simulink model "Privodslx"  (R2022a)
settings: Solver=VariableStepAuto  StartTime=0.0  StopTime=inf  FixedStep=0.01  RelTol=1e-3
undefined symbols (not defined in the file): diff, eul2tform, get, hot, Levenberg, Marquardt, maxWaypoints, q0, traectory, trvec2tform, ts, waypointTimes, X, Y, Z
libraries: sm_lib x250, nesl_utility x51, trajExampleUtils x23, robotcorelib x19, robotmaniplib x5, Contact_Forces_Lib x1, dspobslib x1
(part 1 of 6)
settings Model: Creator=tystr  LastModifiedBy=tystr
settings SolverCC: AlgebraicLoopSolver=TrustRegion
settings DebuggingCC: ReadBeforeWriteMsg=DisableAll  WriteAfterWriteMsg=DisableAll  WriteAfterReadMsg=DisableAll  MultiTaskDSMMsg=none  UnconnectedInputMsg=warning  UnconnectedOutputMsg=warning  UnconnectedLineMsg=warning  SFMachineParentedDataDiag=warning
settings SFSimCC: CustomCodeUndefinedFunction=UseInterfaceOnly
settings RTWCC: DLArmComputeVersion=19.05
settings ExplorerConfigSet: InternalSimMechanicsExplorerSettings="<ExplorerConfiguration><canonicalview>default</canonicalview><AnimationSetting><BasePlaybackSpeed>1.0</BasePlaybackSpeed><PlaybackSpeedFactor>1.0</PlaybackSpeedFactor></AnimationSetting><TilePanel><TileInfo><Tiles Columns=\"1\" Count=\"1\" Rows=\"1\"><Column Weight=\"1\"/><Row Weight=\"1\"/><Tile Height=\"1\" Width=\"1\" X=\"0\" Y=\"0\"/></Tiles></TileInfo><SceneInfo><SceneViewer><BGColor><R>0.800000011920928955</R><G>0.800000011920928955</G><B>0.800000011920928955</B></BGColor><Camera><DoPerspective>off</DoPerspective><Position><X>0.581172870773565831</X><Y>-0.777808712780073574</Y><Z>0.308286162888697479</Z></Position><Center><X>0.305915452038245772</X><Y>0.176306748607351294</Y><Z>0.190400456491913256</Z></Center><Up><X>-0.216141355262336798</X><Y>0.0580651955211244353</Y><Z>0.974633955705655919</Z></Up><ViewLimDist>1</ViewLimDist><YLim>0.905328153776305378</YLim><XLim>1.29865056944726809</XLim></Camera></SceneViewer></SceneInfo></TilePanel><MechEditorPanel><Cameras><Camera><Id>Camera1</Id><Value><Name>Camera1</Name><NativeCamera><PositionTrackingFeature>UR1.tool0.F.frame</PositionTrackingFeature><CenterTrackingFeature>UR1.tool0.F.frame</CenterTrackingFeature><UpVectorTrackingFeature>UR1.tool0.F.frame</UpVectorTrackingFeature><CenterTrackingOrigin>off</CenterTrackingOrigin><CenterTrackingDirection>+Z</CenterTrackingDirection><UpVectorTrackingDirection>-X</UpVectorTrackingDirection></NativeCamera></Value></Camera></Cameras><GfxPanelCameraMap/><VideoCreator><PlaybackSpeedRatio>1.0</PlaybackSpeedRatio><FrameRate>60</FrameRate><VideoFormat>MPEG-4</VideoFormat><FrameSize>[1920 1080]</FrameSize></VideoCreator></MechEditorPanel></ExplorerConfiguration>"

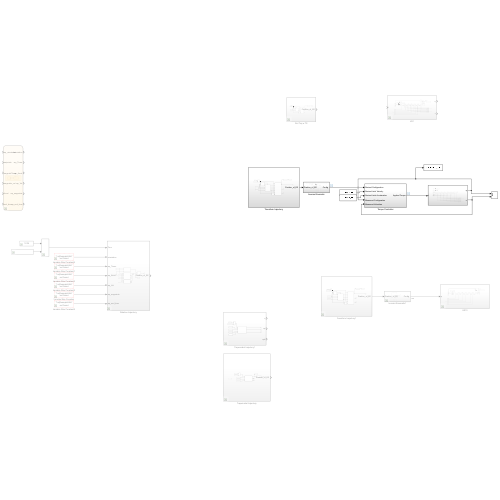
[thumbnail: Simulink's stored preview of the top-level diagram]
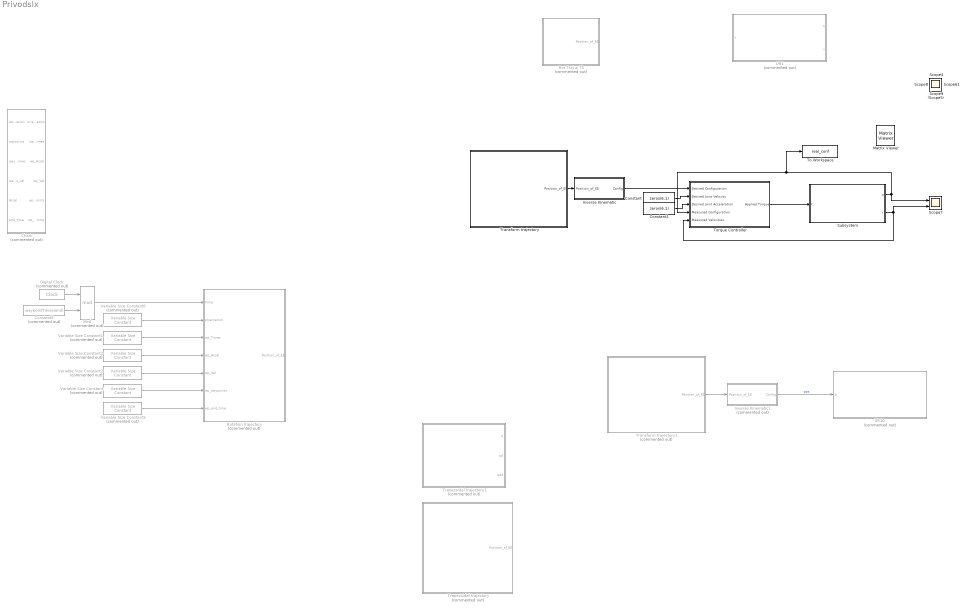
== system Privodslx ==
  Chart : Stateflow chart  Commented=on  TreatAsAtomicUnit=on
      settings: PortSchema="{\"entries\":[{\"content\":{\"sides\":[{\"content\":{\"connectorIds\":[\"In4\",\"In2\",\"In1\",\"In3\",\"In5\",\"In6\"]},\"type\":\"ConnectorPlacement.EquallySpacedRectSide\",\"uuid\":\"199a3ae9-d570-4542-b92b-f36511b0c15c\"},{\"content\":{\"connectorIds\":[\"Out1\",\"Out2\",\"Out3\",\"Out4\",\"Out5\",\"Out6\"],\"side\":\"RIGHT\"},\"type\":\"ConnectorPlacement.EquallySpacedRectSide\",\"uuid\":\"03e9b347-4596-49f5-8d91-254a4ca3c338\"},{\"content\":{\"connectorIds\":[],\"side\":\"TOP\"},\"type\":\"ConnectorPlacement.EquallySpacedRectSide\",\"uuid\":\"99359905-edef-4f33-b514-45af203258c0\"},{\"content\":{\"connectorIds\":[],\"side\":\"HIDDEN\"},\"type\":\"ConnectorPlacement.EquallySpacedRectSide\",\"uuid\":\"67583bbf-e95c-431d-a69b-7f52f21df5ab\"}]},\"type\":\"ConnectorPlacement.EquallySpacedConnector\",\"uuid\":\"4447fce3-df88-4ff0-a93e-6e37d8f328a3\"}],\"packageUris\":[\"http://schema.mathworks.com/mf0/Connector/R2020b\"],\"version\":\"1.0\"}"
  Constant : Constant  Value=zeros(6,1)  SampleTime=0.01
  Constant1 : Constant  Value=zeros(6,1)  SampleTime=0.01
  Constant5 : Constant  Commented=on  Value=waypointTimes(end)
  Digital Clock : DigitalClock  Commented=on  SampleTime=ts
  Inverse Kinematic : Subsystem
  Inverse Kinematic1 : Subsystem  Commented=on
  Mod : Math  Commented=on  Operator=mod  SignedPower=on
  Rot Traj w TS : Subsystem  Commented=on
  Rotation trajectory : Subsystem  Commented=on
  Scope7 : Scope  NumInputPorts=2
  Subsystem : Subsystem
  To Workspace : ToWorkspace  VariableName=real_conf  SaveFormat=Timeseries  SampleTime=-1
  Torque Controller : Subsystem
  Transform trajectory : Subsystem
  Transform trajectory1 : Subsystem  Commented=on
  Trapezoidal trajectory : Subsystem  Commented=on
  Trapezoidal trajectory1 : Subsystem  Commented=on
  UR1 : Subsystem  Commented=on
  UR10 : Subsystem  Commented=on
  Variable Size Constant : trajExampleUtils/Variable Size Constant  Commented=on  val=waypoints  maxSize=[3,maxWaypoints]  Ts=ts  SSRTWFcnClass=[]
  Variable Size Constant1 : trajExampleUtils/Variable Size Constant  Commented=on  val=waypointTimes  maxSize=[1,maxWaypoints]  Ts=ts  SSRTWFcnClass=[]
  Variable Size Constant2 : trajExampleUtils/Variable Size Constant  Commented=on  val=waypointVels  maxSize=[3,maxWaypoints]  Ts=ts  SSRTWFcnClass=[]
  Variable Size Constant3 : trajExampleUtils/Variable Size Constant  Commented=on  val=waypointAccels  maxSize=[3,maxWaypoints]  Ts=ts  SSRTWFcnClass=[]
  Variable Size Constant5 : trajExampleUtils/Variable Size Constant  Commented=on  val=repmat(diff(waypointTimes),[3 1])  maxSize=[3,maxWaypoints-1]  Ts=ts  SSRTWFcnClass=[]
  Variable Size Constant6 : trajExampleUtils/Variable Size Constant  Commented=on  val=orientations  maxSize=[3,maxWaypoints]  Ts=ts  SSRTWFcnClass=[]
  Matrix Viewer : dspobslib/Matrix Viewer  IOType=viewer  ImageParams=off  CMapStr=hot(256)  AxisColorbar=on  AxisParams=off  AxisOrigin=Upper left corner  AxisTickMode=Auto  XTickRange=[0 1]  YTickRange=[0 1]  XLabel=X-axis  YLabel=Y-axis  ZLabel=Z-axis  FigPos=get(0,'defaultfigureposition')  AxisZoom=off
      settings: SourceProductName=DSP System Toolbox  YMin=-1.0  YMax=1.0
  Scope{,1..6,8..11} (11 alike) : Scope
  wires:
  Transform trajectory1/1("Position_of_EE ") -> Inverse Kinematic1/1("Position_of_EE ")
  Inverse Kinematic1/1("Config ") -> UR10/1(q)  "pos"
  Constant1/1 -> Torque Controller/3(Desired Joint Acceleration)
  Digital Clock/1 -> Mod/1
  Constant5/1 -> Mod/2
  Mod/1 -> Rotation trajectory/1(Time)
  Variable Size Constant6/1 -> Rotation trajectory/2(orientation)
  Variable Size Constant/1 -> Rotation trajectory/6(wp_waypoints)
  Variable Size Constant1/1 -> Rotation trajectory/3(wp_Times)
  Variable Size Constant2/1 -> Rotation trajectory/5(wp_Vel)
  Variable Size Constant3/1 -> Rotation trajectory/4(wp_Accel)
  Variable Size Constant5/1 -> Rotation trajectory/7(wp_end_time)
  Constant/1 -> Torque Controller/2(Desired Joint Velocity)
  Transform trajectory/1("Position_of_EE ") -> Inverse Kinematic/1("Position_of_EE ")
  Subsystem/1(q) -> Scope7/1, To Workspace/1, Torque Controller/4(Measured Configuration)
  Subsystem/2(v) -> Torque Controller/5(Measured Velocities), Scope7/2
  Torque Controller/1(Applied Torque) -> Subsystem/1(t)
  Inverse Kinematic/1("Config ") -> Torque Controller/1(Desired Configuration)

== system Privodslx/Inverse Kinematic ==
  "Position_of_EE " : Inport  SampleTime=ts
  Bus Selector : BusSelector  Commented=on  OutputSignals=Iterations,PoseErrorNorm,ExitFlag,Status
  Constant : Constant  Value=[1,1,1,1,1,1]
  Delay : Delay  DelayLength=1  InitialCondition=q0  SampleTime=ts
  Display{3..6} (4 alike) : Display  Commented=on
  Inverse Kinematics : robotmaniplib/Inverse Kinematics  RigidBodyTree=robot  EndEffector=tool0  ShowInfo=on  SolverName=Levenberg-Marquardt  EnforceJointLimits=on  MaxIterations=1500  MaxTime=10  GradientTolerance=1e-7  SolutionTolerance=1e-6  StepTolerance=1e-14  ErrorChangeTolerance=1e-12  UseErrorDamping=on  DampingBias=0.0025  SimulateUsing=Interpreted execution
  To Workspace : ToWorkspace  VariableName=config  SaveFormat=Timeseries  SampleTime=-1
  To Workspace1 : ToWorkspace  VariableName=info  SaveFormat=Timeseries  SampleTime=-1
  "Config " : Outport  SampleTime=ts  VectorParamsAs1DForOutWhenUnconnected=off
  wires:
  Bus Selector/3 -> Display5/1  "<ExitFlag>"
  Inverse Kinematics/1 -> Delay/1, To Workspace/1, "Config "/1
  Bus Selector/4 -> Display6/1  "<Status>"
  Inverse Kinematics/2 -> To Workspace1/1
  Bus Selector/2 -> Display4/1  "<PoseErrorNorm>"
  "Position_of_EE "/1 -> Inverse Kinematics/1
  Constant/1 -> Inverse Kinematics/2
  Bus Selector/1 -> Display3/1  "<Iterations>"
  Delay/1 -> Inverse Kinematics/3

== system Privodslx/Inverse Kinematic1 ==
  "Position_of_EE " : Inport
  Bus Selector : BusSelector  Commented=on  OutputSignals=Iterations,PoseErrorNorm,ExitFlag,Status
  Constant : Constant  Value=[1,1,1,1,1,1]
  Delay : Delay  DelayLength=1  InitialCondition=zeros(6,1)
  Display : Display
  Display{3..6} (4 alike) : Display  Commented=on
  Inverse Kinematics1 : robotmaniplib/Inverse Kinematics  RigidBodyTree=robot  EndEffector=tool0  ShowInfo=on  SolverName=Levenberg-Marquardt  EnforceJointLimits=off  MaxIterations=1500  MaxTime=10  GradientTolerance=1e-7  SolutionTolerance=1e-6  StepTolerance=1e-14  ErrorChangeTolerance=1e-12  UseErrorDamping=on  DampingBias=0.0025  SimulateUsing=Interpreted execution
  Scope : Scope
  To Workspace : ToWorkspace  VariableName=config  SaveFormat=Timeseries  SampleTime=-1
  To Workspace1 : ToWorkspace  VariableName=info  SaveFormat=Timeseries  SampleTime=-1
  "Config " : Outport  VectorParamsAs1DForOutWhenUnconnected=off
  wires:
  Bus Selector/1 -> Display3/1  "<Iterations>"
  Constant/1 -> Inverse Kinematics1/2
  "Position_of_EE "/1 -> Inverse Kinematics1/1, Display/1
  Delay/1 -> Inverse Kinematics1/3
  Bus Selector/2 -> Display4/1  "<PoseErrorNorm>"
  Inverse Kinematics1/2 -> To Workspace1/1
  Bus Selector/4 -> Display6/1  "<Status>"
  Inverse Kinematics1/1 -> Delay/1, "Config "/1, Scope/1, To Workspace/1
  Bus Selector/3 -> Display5/1  "<ExitFlag>"

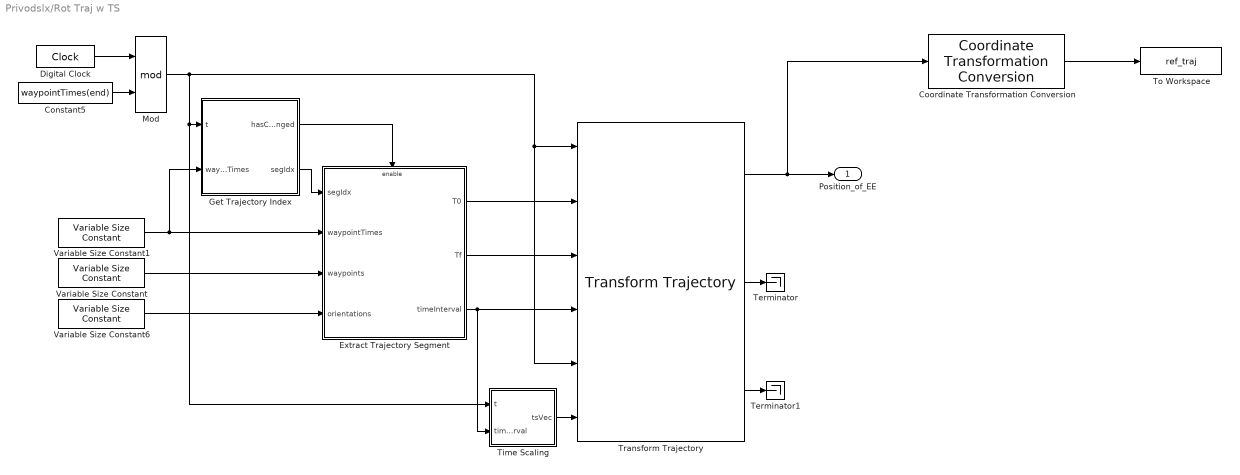
== system Privodslx/Rot Traj w TS ==
  Constant5 : Constant  Value=waypointTimes(end)
  Coordinate Transformation Conversion : robotcorelib/Coordinate Transformation Conversion  InputRepresentation=Homogeneous Transformation  InputEulerSequence=ZYX  ShowTrVecInputPort=on  OutputRepresentation=Translation Vector  OutputEulerSequence=ZYX  ShowTrVecOutputPort=on  SimulateUsing=Interpreted execution
      settings: SourceProductBaseCode=RO,NV,RR,UV
  Digital Clock : DigitalClock  SampleTime=ts
  Extract Trajectory Segment : Subsystem
  Get Trajectory Index : MATLAB Function  TreatAsAtomicUnit=on
  Mod : Math  Operator=mod  SignedPower=on
  Terminator : Terminator
  Terminator1 : Terminator
  Time Scaling : Subsystem
  To Workspace : ToWorkspace  VariableName=ref_traj  SaveFormat=Timeseries  SampleTime=-1
  Transform Trajectory : robotcorelib/Transform Trajectory  WaypointSource=External  T0=trvec2tform( [ 1, 10, -1 ] )  TF=eul2tform( [ 0, pi, pi / 2 ] )  TimeInterval=[ 2, 3 ]  CustomTimeScaling=on  ParameterSource=External  TSTime=2:0.1:3  TimeScaling=[ 0:0.1:1; ones( 1, 11 ); zeros( 1, 11 ) ]  SimulateUsing=Interpreted execution
      settings: SourceProductBaseCode=RO,NV,RR,UV
  Variable Size Constant : trajExampleUtils/Variable Size Constant  val=waypoints  maxSize=[3,maxWaypoints]  Ts=-1
  Variable Size Constant1 : trajExampleUtils/Variable Size Constant  val=waypointTimes  maxSize=[1,maxWaypoints]  Ts=-1
  Variable Size Constant6 : trajExampleUtils/Variable Size Constant  val=orientations  maxSize=[3,maxWaypoints]  Ts=-1
  "Position_of_EE " : Outport
  wires:
  Variable Size Constant1/1 -> Extract Trajectory Segment/2(waypointTimes), Get Trajectory Index/2(waypointTimes)
  Transform Trajectory/2 -> Terminator/1
  Variable Size Constant6/1 -> Extract Trajectory Segment/4(orientations)
  Time Scaling/1(tsVec) -> Transform Trajectory/6
  Mod/1 -> Transform Trajectory/1, Transform Trajectory/5, Time Scaling/1(t), Get Trajectory Index/1(t)
  Extract Trajectory Segment/3(timeInterval) -> Transform Trajectory/4, Time Scaling/2(timeInterval)
  Extract Trajectory Segment/2(Tf) -> Transform Trajectory/3
  Get Trajectory Index/2(segIdx) -> Extract Trajectory Segment/1(segIdx)
  Extract Trajectory Segment/1(T0) -> Transform Trajectory/2
  Get Trajectory Index/1(hasChanged) -> Extract Trajectory Segment/Enable
  Transform Trajectory/3 -> Terminator1/1
  Variable Size Constant/1 -> Extract Trajectory Segment/3(waypoints)
  Digital Clock/1 -> Mod/1
  Constant5/1 -> Mod/2
  Transform Trajectory/1 -> Coordinate Transformation Conversion/1, "Position_of_EE "/1
  Coordinate Transformation Conversion/1 -> To Workspace/1

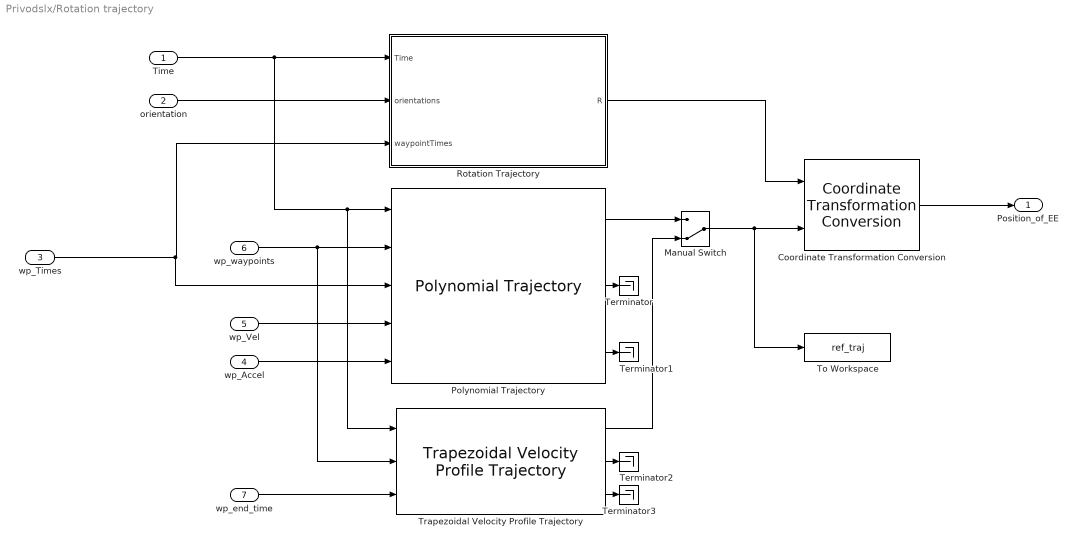
== system Privodslx/Rotation trajectory ==
  Time : Inport
  orientation : Inport  Port=2
  wp_Times : Inport  Port=3
  wp_Accel : Inport  Port=4
  wp_Vel : Inport  Port=5
  wp_waypoints : Inport  Port=6
  wp_end_time : Inport  Port=7
  Coordinate Transformation Conversion : robotcorelib/Coordinate Transformation Conversion  InputRepresentation=Quaternion  InputEulerSequence=ZYX  ShowTrVecInputPort=on  OutputRepresentation=Homogeneous Transformation  OutputEulerSequence=ZYX  ShowTrVecOutputPort=on  SimulateUsing=Interpreted execution
      settings: SourceProductBaseCode=RO,NV,RR,UV
  Manual Switch : ManualSwitch  CurrentSetting=0
  Polynomial Trajectory : robotcorelib/Polynomial Trajectory  WaypointSource=External  Waypoints=[ 0, 2, 1, 5, 0; -1, 3, 1, 4, 4 ]  TimePoints=[ 0, 1, 2, 3, 4 ]  TimeInterval=[ 1, 4 ]  Method=Quintic Polynomial  ParameterSource=External  VelocityBoundaryCondition=zeros( 2, 5 )  AccelerationBoundaryCondition=zeros( 2, 5 )  SimulateUsing=Interpreted execution
      settings: SourceProductBaseCode=RO,NV,RR,UV
  Rotation Trajectory : Subsystem
  Terminator{,1..3} (4 alike) : Terminator
  To Workspace : ToWorkspace  VariableName=ref_traj  SaveFormat=Timeseries  SampleTime=-1
  Trapezoidal Velocity Profile Trajectory : robotcorelib/Trapezoidal Velocity Profile Trajectory  WaypointSource=External  Waypoints=[ 0, -0.5, -1; 0, 0.5, 1 ]  NumParams=1  Parameter1=End Time  Parameter2=End Time  ParameterSource=External  PeakVelocity=[ 1; 1; 1 ]  Acceleration=[ 1; 2 ]  EndTime=[ 1; 1; 1 ]  AccelTime=[ 1; 2 ]  SimulateUsing=Interpreted execution
      settings: SourceProductBaseCode=RO,NV,RR,UV
  "Position_of_EE " : Outport  SampleTime=ts
  wires:
  Manual Switch/1 -> To Workspace/1, Coordinate Transformation Conversion/2
  Polynomial Trajectory/1 -> Manual Switch/1
  Trapezoidal Velocity Profile Trajectory/2 -> Terminator2/1
  Rotation Trajectory/1(R) -> Coordinate Transformation Conversion/1
  Trapezoidal Velocity Profile Trajectory/3 -> Terminator3/1
  Trapezoidal Velocity Profile Trajectory/1 -> Manual Switch/2
  Polynomial Trajectory/3 -> Terminator1/1
  Polynomial Trajectory/2 -> Terminator/1
  Coordinate Transformation Conversion/1 -> "Position_of_EE "/1
  Time/1 -> Trapezoidal Velocity Profile Trajectory/1, Polynomial Trajectory/1, Rotation Trajectory/1(Time)
  orientation/1 -> Rotation Trajectory/2(orientations)
  wp_Times/1 -> Polynomial Trajectory/3, Rotation Trajectory/3(waypointTimes)
  wp_Accel/1 -> Polynomial Trajectory/5
  wp_Vel/1 -> Polynomial Trajectory/4
  wp_waypoints/1 -> Trapezoidal Velocity Profile Trajectory/2, Polynomial Trajectory/2
  wp_end_time/1 -> Trapezoidal Velocity Profile Trajectory/3

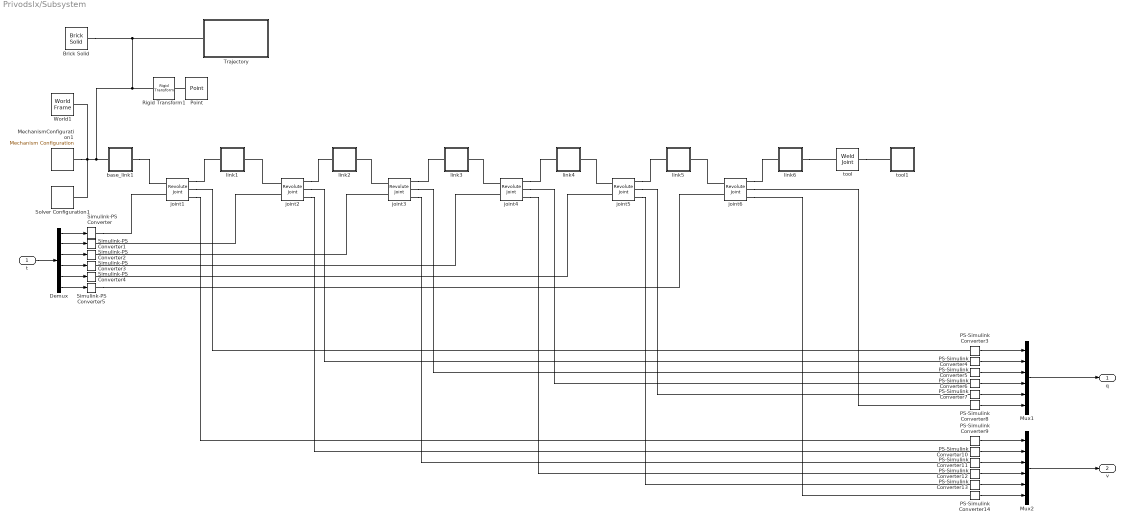
== system Privodslx/Subsystem ==
  t : Inport  SampleTime=ts
  Brick Solid : sm_lib/Body Elements/Brick Solid  GraphicAmbientColor=[0.15 0.15 0.15 1.0]  BasedOnType=Density  BrickDimensions=[1.5 1.5 0.01]  BrickDimensionUnits=m  CenterOfMass=[0 0 0]  CenterOfMassUnits=m  GraphicDiffuseColor=[0.5019608 0.72156864 0.3019608]  Density=1000  DensityUnits=kg/m^3  DoExposeReferenceFrame=on  GraphicEmissiveColor=[0.0 0.0 0.0 1.0]  ExportEntireGeometry=off  SerializedFrames=<Frames/>  MarkerShape=Sphere  MarkerSize=10  GraphicType=FromGeometry  InertiaType=CalculateFromGeometry  Mass=1  MassUnits=kg  MomentsOfInertia=[1 1 1]  MomentsOfInertiaUnits=kg*m^2  GraphicOpacity=1.0  ProductsOfInertia=[0 0 0]  ProductsOfInertiaUnits=kg*m^2  GraphicShininess=75  GraphicSpecularColor=[0.5 0.5 0.5 1.0]  GraphicVisPropType=SimpleVisualProperties
  Demux : Demux  Outputs=6
  MechanismConfiguration1 : sm_lib/Utilities/Mechanism Configuration  UniformGravity=Constant  GravityVector=[0 0 -9.80665]  GravityUnits=m/s^2  LinearizationDelta=0.001  JointModeTransitionNonlinearIterations=2
  Mux1 : Mux  Inputs=6
  Mux2 : Mux  Inputs=6
  PS-Simulink Converter{3..14} (12 alike) : nesl_utility/PS-Simulink Converter  PhysicalDomain=network_engine_domain  SubClassName=ps_output  LeftPortType=input  RightPortType=output  PseudoPeriodic=off  Frequencies=[]  VectorFormat=1-D array  Unit=inherit  AffineConversion=off
      settings: SourceProductBaseCode=SS,PW,VE
  Point : sm_lib/Curves and Surfaces/Point  GraphicType=Marker  MarkerShape=Sphere  MarkerSize=10  GraphicVisPropType=SimpleVisualProperties  GraphicDiffuseColor=[0.5 0.5 0.5]  GraphicOpacity=1.0  GraphicSpecularColor=[0.5 0.5 0.5 1.0]  GraphicAmbientColor=[0.15 0.15 0.15 1.0]  GraphicEmissiveColor=[0.0 0.0 0.0 1.0]  GraphicShininess=75
      settings: SourceProductBaseCode=MS
  Rigid Transform1 : sm_lib/Frames and Transforms/Rigid Transform  TranslationMethod=Cartesian  TranslationStandardOffset=0  TranslationLengthUnit=m  TranslationStandardAxis=+Z  TranslationCartesianOffset=start_vec  TranslationROffset=0  TranslationROffsetUnits=m  TranslationZOffset=0  TranslationZOffsetUnits=m  TranslationThetaOffset=0  TranslationThetaOffsetUnits=deg  RotationMethod=None  RotationAngleUnits=deg  RotationStandardAxis=+Z  RotationAngle=0.0  RotationArbitraryAxis=[0 0 1]  FollAlignAxisA=+X  BaseAlignAxisA=+Y  FollAlignAxisB=+Y  BaseAlignAxisB=+Z  RotationSequenceAxes=FollowerAxes  RotationSequence=XYX  RotationSequenceAngles=[0 0 0]  RotationSequenceAnglesUnits=deg  RotationMatrix=[1 0 0; 0 1 0; 0 0 1]
  Simulink-PS Converter{,1..5} (6 alike) : nesl_utility/Simulink-PS Converter  PhysicalDomain=network_engine_domain  SubClassName=ps_input  LeftPortType=input  RightPortType=output  PseudoPeriodic=off  Frequencies=[]  NoiseDistribution=none  NoiseParameters=[]  Unit=1  AffineConversion=off  FilteringAndDerivatives=provide  SimscapeFilterOrder=2  InputFilterTimeConstant=0.001  UdotUserProvided=0
      settings: SourceProductBaseCode=SS,PW,VE
  Solver Configuration1 : nesl_utility/Solver Configuration  PhysicalDomain=network_engine_domain  SubClassName=solver  LeftPortType=input  RightPortType=generic  Tones=[]  Harmonics=[]  SimulateNoise=off  Profile=off  UseLocalSampling=off  EnableSwitchedLinearOptims=on  FrequencyDomain=off  UseCCode=off  RelTol=0.001  AbsTol=0.001  MinStep=1e-09  ToWorkspace=off  RevertToSquareIcSolve=off  NumHomotopyIterations=100  PhasorMode=off  PhasorModeNumHarmonics=1  IndexReductionMethod=DerivativeReplacement  DoDC=off  ResidualTolerance=1e-09  UseLocalSolver=off  LocalSolverChoice=NE_BACKWARD_EULER_ADVANCER  LocalSolverSampleTime=0.001  DoFixedCost=off  MaxNonlinIter=3  MaxModeIter=2  ComputeImpulses=off  ImpulseIterations=2  LinearAlgebra=auto  LinearAlgebraNumThread=0  EquationFormulation=NE_TIME_EF  DelaysMemoryBudget=1024  AutomaticFiltering=on  FilteringTimeConstant=0.001  PartitionStorageMethod=AS_NEEDED  PartitionMemoryBudget=1024  PartitionMethod=ROBUST
      settings: SourceProductBaseCode=SS,PW,VE
  Trajectory : Subsystem
  World1 : sm_lib/Frames and Transforms/World Frame
  base_link1 : Subsystem
  joint1 : sm_lib/Joints/Revolute Joint  JointMode=Normal  SenseConstraintForce=off  SenseConstraintForceX=off  SenseConstraintForceY=off  SenseConstraintForceZ=off  SenseConstraintTorque=off  SenseConstraintTorqueX=off  SenseConstraintTorqueY=off  SenseConstraintTorqueZ=off  SenseTotalForce=off  SenseTotalForceX=off  SenseTotalForceY=off  SenseTotalForceZ=off  SenseTotalTorque=off  SenseTotalTorqueX=off  SenseTotalTorqueY=off  SenseTotalTorqueZ=off  CompositeWrenchDir=FollowerOnBase  CompositeWrenchFrame=BaseFrame  EquilibriumPosition=0  EquilibriumPositionUnits=deg  SpringStiffness=0  SpringStiffnessUnits=N*m/deg  DampingCoefficient=0  DampingCoefficientUnits=kg*m^2/(rad*s)  TorqueActuationMode=InputTorque  MotionActuationMode=ComputedMotion  SensePosition=on  SenseVelocity=on  SenseAcceleration=off  SenseTorqueForce=off  SenseLowerLimitTorqueForce=off  SenseUpperLimitTorqueForce=off  LowerLimitSpecify=on  LowerLimitBound=-3.1416  LowerLimitBoundUnits=rad  LowerLimitStiffness=1e4  LowerLimitStiffnessUnits=N*m/deg  LowerLimitDamping=10  LowerLimitDampingUnits=N*m/(deg/s)  LowerLimitTransitionRegionWidth=0.1  LowerLimitTransitionRegionWidthUnits=deg  UpperLimitSpecify=on  UpperLimitBound=3.1416  UpperLimitBoundUnits=rad  UpperLimitStiffness=1e4  UpperLimitStiffnessUnits=N*m/deg  UpperLimitDamping=10  UpperLimitDampingUnits=N*m/(deg/s)  UpperLimitTransitionRegionWidth=0.1  UpperLimitTransitionRegionWidthUnits=deg  PositionTargetSpecify=off  PositionTargetPriority=High  PositionTargetValue=0  PositionTargetValueUnits=deg  VelocityTargetSpecify=off  VelocityTargetPriority=High  VelocityTargetValue=0  VelocityTargetValueUnits=deg/s
  joint2 : sm_lib/Joints/Revolute Joint  JointMode=Normal  SenseConstraintForce=off  SenseConstraintForceX=off  SenseConstraintForceY=off  SenseConstraintForceZ=off  SenseConstraintTorque=off  SenseConstraintTorqueX=off  SenseConstraintTorqueY=off  SenseConstraintTorqueZ=off  SenseTotalForce=off  SenseTotalForceX=off  SenseTotalForceY=off  SenseTotalForceZ=off  SenseTotalTorque=off  SenseTotalTorqueX=off  SenseTotalTorqueY=off  SenseTotalTorqueZ=off  CompositeWrenchDir=FollowerOnBase  CompositeWrenchFrame=BaseFrame  EquilibriumPosition=0  EquilibriumPositionUnits=deg  SpringStiffness=0  SpringStiffnessUnits=N*m/deg  DampingCoefficient=0  DampingCoefficientUnits=kg*m^2/(rad*s)  TorqueActuationMode=InputTorque  MotionActuationMode=ComputedMotion  SensePosition=on  SenseVelocity=on  SenseAcceleration=off  SenseTorqueForce=off  SenseLowerLimitTorqueForce=off  SenseUpperLimitTorqueForce=off  LowerLimitSpecify=on  LowerLimitBound=-1.5708  LowerLimitBoundUnits=rad  LowerLimitStiffness=1e4  LowerLimitStiffnessUnits=N*m/deg  LowerLimitDamping=10  LowerLimitDampingUnits=N*m/(deg/s)  LowerLimitTransitionRegionWidth=0.1  LowerLimitTransitionRegionWidthUnits=deg  UpperLimitSpecify=on  UpperLimitBound=3.1415  UpperLimitBoundUnits=rad  UpperLimitStiffness=1e4  UpperLimitStiffnessUnits=N*m/deg  UpperLimitDamping=10  UpperLimitDampingUnits=N*m/(deg/s)  UpperLimitTransitionRegionWidth=0.1  UpperLimitTransitionRegionWidthUnits=deg  PositionTargetSpecify=off  PositionTargetPriority=High  PositionTargetValue=0  PositionTargetValueUnits=deg  VelocityTargetSpecify=off  VelocityTargetPriority=High  VelocityTargetValue=0  VelocityTargetValueUnits=deg/s
  joint3 : sm_lib/Joints/Revolute Joint  JointMode=Normal  SenseConstraintForce=off  SenseConstraintForceX=off  SenseConstraintForceY=off  SenseConstraintForceZ=off  SenseConstraintTorque=off  SenseConstraintTorqueX=off  SenseConstraintTorqueY=off  SenseConstraintTorqueZ=off  SenseTotalForce=off  SenseTotalForceX=off  SenseTotalForceY=off  SenseTotalForceZ=off  SenseTotalTorque=off  SenseTotalTorqueX=off  SenseTotalTorqueY=off  SenseTotalTorqueZ=off  CompositeWrenchDir=FollowerOnBase  CompositeWrenchFrame=BaseFrame  EquilibriumPosition=0  EquilibriumPositionUnits=deg  SpringStiffness=0  SpringStiffnessUnits=N*m/deg  DampingCoefficient=0  DampingCoefficientUnits=kg*m^2/(rad*s)  TorqueActuationMode=InputTorque  MotionActuationMode=ComputedMotion  SensePosition=on  SenseVelocity=on  SenseAcceleration=off  SenseTorqueForce=off  SenseLowerLimitTorqueForce=off  SenseUpperLimitTorqueForce=off  LowerLimitSpecify=on  LowerLimitBound=-3.1416  LowerLimitBoundUnits=rad  LowerLimitStiffness=1e4  LowerLimitStiffnessUnits=N*m/deg  LowerLimitDamping=10  LowerLimitDampingUnits=N*m/(deg/s)  LowerLimitTransitionRegionWidth=0.1  LowerLimitTransitionRegionWidthUnits=deg  UpperLimitSpecify=on  UpperLimitBound=3.1416  UpperLimitBoundUnits=rad  UpperLimitStiffness=1e4  UpperLimitStiffnessUnits=N*m/deg  UpperLimitDamping=10  UpperLimitDampingUnits=N*m/(deg/s)  UpperLimitTransitionRegionWidth=0.1  UpperLimitTransitionRegionWidthUnits=deg  PositionTargetSpecify=off  PositionTargetPriority=High  PositionTargetValue=0  PositionTargetValueUnits=deg  VelocityTargetSpecify=off  VelocityTargetPriority=High  VelocityTargetValue=0  VelocityTargetValueUnits=deg/s
  joint4 : sm_lib/Joints/Revolute Joint  JointMode=Normal  SenseConstraintForce=off  SenseConstraintForceX=off  SenseConstraintForceY=off  SenseConstraintForceZ=off  SenseConstraintTorque=off  SenseConstraintTorqueX=off  SenseConstraintTorqueY=off  SenseConstraintTorqueZ=off  SenseTotalForce=off  SenseTotalForceX=off  SenseTotalForceY=off  SenseTotalForceZ=off  SenseTotalTorque=off  SenseTotalTorqueX=off  SenseTotalTorqueY=off  SenseTotalTorqueZ=off  CompositeWrenchDir=FollowerOnBase  CompositeWrenchFrame=BaseFrame  EquilibriumPosition=0  EquilibriumPositionUnits=deg  SpringStiffness=0  SpringStiffnessUnits=N*m/deg  DampingCoefficient=0  DampingCoefficientUnits=kg*m^2/(rad*s)  TorqueActuationMode=InputTorque  MotionActuationMode=ComputedMotion  SensePosition=on  SenseVelocity=on  SenseAcceleration=off  SenseTorqueForce=off  SenseLowerLimitTorqueForce=off  SenseUpperLimitTorqueForce=off  LowerLimitSpecify=on  LowerLimitBound=-1.5708  LowerLimitBoundUnits=rad  LowerLimitStiffness=1e4  LowerLimitStiffnessUnits=N*m/deg  LowerLimitDamping=10  LowerLimitDampingUnits=N*m/(deg/s)  LowerLimitTransitionRegionWidth=0.1  LowerLimitTransitionRegionWidthUnits=deg  UpperLimitSpecify=on  UpperLimitBound=3.1416  UpperLimitBoundUnits=rad  UpperLimitStiffness=1e4  UpperLimitStiffnessUnits=N*m/deg  UpperLimitDamping=10  UpperLimitDampingUnits=N*m/(deg/s)  UpperLimitTransitionRegionWidth=0.1  UpperLimitTransitionRegionWidthUnits=deg  PositionTargetSpecify=off  PositionTargetPriority=High  PositionTargetValue=0  PositionTargetValueUnits=deg  VelocityTargetSpecify=off  VelocityTargetPriority=High  VelocityTargetValue=0  VelocityTargetValueUnits=deg/s
  joint5 : sm_lib/Joints/Revolute Joint  JointMode=Normal  SenseConstraintForce=off  SenseConstraintForceX=off  SenseConstraintForceY=off  SenseConstraintForceZ=off  SenseConstraintTorque=off  SenseConstraintTorqueX=off  SenseConstraintTorqueY=off  SenseConstraintTorqueZ=off  SenseTotalForce=off  SenseTotalForceX=off  SenseTotalForceY=off  SenseTotalForceZ=off  SenseTotalTorque=off  SenseTotalTorqueX=off  SenseTotalTorqueY=off  SenseTotalTorqueZ=off  CompositeWrenchDir=FollowerOnBase  CompositeWrenchFrame=BaseFrame  EquilibriumPosition=0  EquilibriumPositionUnits=deg  SpringStiffness=0  SpringStiffnessUnits=N*m/deg  DampingCoefficient=0  DampingCoefficientUnits=kg*m^2/(rad*s)  TorqueActuationMode=InputTorque  MotionActuationMode=ComputedMotion  SensePosition=on  SenseVelocity=on  SenseAcceleration=off  SenseTorqueForce=off  SenseLowerLimitTorqueForce=off  SenseUpperLimitTorqueForce=off  LowerLimitSpecify=on  LowerLimitBound=-3.1416  LowerLimitBoundUnits=rad  LowerLimitStiffness=1e4  LowerLimitStiffnessUnits=N*m/deg  LowerLimitDamping=10  LowerLimitDampingUnits=N*m/(deg/s)  LowerLimitTransitionRegionWidth=0.1  LowerLimitTransitionRegionWidthUnits=deg  UpperLimitSpecify=on  UpperLimitBound=3.1416  UpperLimitBoundUnits=rad  UpperLimitStiffness=1e4  UpperLimitStiffnessUnits=N*m/deg  UpperLimitDamping=10  UpperLimitDampingUnits=N*m/(deg/s)  UpperLimitTransitionRegionWidth=0.1  UpperLimitTransitionRegionWidthUnits=deg  PositionTargetSpecify=off  PositionTargetPriority=High  PositionTargetValue=0  PositionTargetValueUnits=deg  VelocityTargetSpecify=off  VelocityTargetPriority=High  VelocityTargetValue=0  VelocityTargetValueUnits=deg/s
  joint6 : sm_lib/Joints/Revolute Joint  JointMode=Normal  SenseConstraintForce=off  SenseConstraintForceX=off  SenseConstraintForceY=off  SenseConstraintForceZ=off  SenseConstraintTorque=off  SenseConstraintTorqueX=off  SenseConstraintTorqueY=off  SenseConstraintTorqueZ=off  SenseTotalForce=off  SenseTotalForceX=off  SenseTotalForceY=off  SenseTotalForceZ=off  SenseTotalTorque=off  SenseTotalTorqueX=off  SenseTotalTorqueY=off  SenseTotalTorqueZ=off  CompositeWrenchDir=FollowerOnBase  CompositeWrenchFrame=BaseFrame  EquilibriumPosition=0  EquilibriumPositionUnits=deg  SpringStiffness=0  SpringStiffnessUnits=N*m/deg  DampingCoefficient=0  DampingCoefficientUnits=kg*m^2/(rad*s)  TorqueActuationMode=InputTorque  MotionActuationMode=ComputedMotion  SensePosition=on  SenseVelocity=on  SenseAcceleration=off  SenseTorqueForce=off  SenseLowerLimitTorqueForce=off  SenseUpperLimitTorqueForce=off  LowerLimitSpecify=on  LowerLimitBound=-1.5708  LowerLimitBoundUnits=rad  LowerLimitStiffness=1e4  LowerLimitStiffnessUnits=N*m/deg  LowerLimitDamping=10  LowerLimitDampingUnits=N*m/(deg/s)  LowerLimitTransitionRegionWidth=0.1  LowerLimitTransitionRegionWidthUnits=deg  UpperLimitSpecify=on  UpperLimitBound=3.1416  UpperLimitBoundUnits=rad  UpperLimitStiffness=1e4  UpperLimitStiffnessUnits=N*m/deg  UpperLimitDamping=10  UpperLimitDampingUnits=N*m/(deg/s)  UpperLimitTransitionRegionWidth=0.1  UpperLimitTransitionRegionWidthUnits=deg  PositionTargetSpecify=off  PositionTargetPriority=High  PositionTargetValue=0  PositionTargetValueUnits=deg  VelocityTargetSpecify=off  VelocityTargetPriority=High  VelocityTargetValue=0  VelocityTargetValueUnits=deg/s
  link1 : Subsystem
  link2 : Subsystem
  link3 : Subsystem
  link4 : Subsystem
  link5 : Subsystem
  link6 : Subsystem
  tool : sm_lib/Joints/Weld Joint  JointMode=Normal  SenseConstraintForce=off  SenseConstraintForceX=off  SenseConstraintForceY=off  SenseConstraintForceZ=off  SenseConstraintTorque=off  SenseConstraintTorqueX=off  SenseConstraintTorqueY=off  SenseConstraintTorqueZ=off  SenseTotalForce=off  SenseTotalForceX=off  SenseTotalForceY=off  SenseTotalForceZ=off  SenseTotalTorque=off  SenseTotalTorqueX=off  SenseTotalTorqueY=off  SenseTotalTorqueZ=off  CompositeWrenchDir=FollowerOnBase  CompositeWrenchFrame=BaseFrame
  tool1 : Subsystem
  q : Outport  SampleTime=ts
  v : Outport  Port=2  SampleTime=ts
  wires:
  PS-Simulink Converter5/1 -> Mux1/3
  Demux/2 -> Simulink-PS Converter1/1
  PS-Simulink Converter13/1 -> Mux2/5
  Mux1/1 -> q/1
  Mux2/1 -> v/1
  Demux/6 -> Simulink-PS Converter5/1
  Demux/4 -> Simulink-PS Converter3/1
  Demux/5 -> Simulink-PS Converter4/1
  PS-Simulink Converter8/1 -> Mux1/6
  Demux/3 -> Simulink-PS Converter2/1
  PS-Simulink Converter3/1 -> Mux1/1
  PS-Simulink Converter7/1 -> Mux1/5
  PS-Simulink Converter6/1 -> Mux1/4
  Demux/1 -> Simulink-PS Converter/1
  PS-Simulink Converter11/1 -> Mux2/3
  PS-Simulink Converter12/1 -> Mux2/4
  PS-Simulink Converter9/1 -> Mux2/1
  PS-Simulink Converter14/1 -> Mux2/6
  PS-Simulink Converter10/1 -> Mux2/2
  t/1 -> Demux/1
  PS-Simulink Converter4/1 -> Mux1/2
  connections:
  Point/LConn1 -- Rigid Transform1/RConn1
  Brick Solid/RConn1 -- base_link1/LConn1 -- World1/RConn1 -- MechanismConfiguration1/RConn1 -- Solver Configuration1/RConn1 -- Rigid Transform1/LConn1 -- Trajectory/LConn1
  joint3/RConn1 -- link3/LConn1
  joint5/LConn1 -- link4/RConn1
  joint5/RConn1 -- link5/LConn1
  joint4/RConn1 -- link4/LConn1
  joint6/RConn1 -- link6/LConn1
  joint4/LConn1 -- link3/RConn1
  joint2/RConn1 -- link2/LConn1
  joint3/LConn1 -- link2/RConn1
  tool/RConn1 -- tool1/LConn1
  joint6/LConn1 -- link5/RConn1
  link6/RConn1 -- tool/LConn1
  joint2/LConn1 -- link1/RConn1
  joint1/RConn1 -- link1/LConn1
  base_link1/RConn1 -- joint1/LConn1
  Simulink-PS Converter/RConn1 -- joint1/LConn2
  Simulink-PS Converter1/RConn1 -- joint2/LConn2
  Simulink-PS Converter2/RConn1 -- joint3/LConn2
  Simulink-PS Converter3/RConn1 -- joint4/LConn2
  Simulink-PS Converter4/RConn1 -- joint5/LConn2
  Simulink-PS Converter5/RConn1 -- joint6/LConn2
  joint1/RConn2 -- PS-Simulink Converter3/LConn1
  joint2/RConn2 -- PS-Simulink Converter4/LConn1
  joint3/RConn2 -- PS-Simulink Converter5/LConn1
  joint4/RConn2 -- PS-Simulink Converter6/LConn1
  joint5/RConn2 -- PS-Simulink Converter7/LConn1
  joint6/RConn2 -- PS-Simulink Converter8/LConn1
  joint1/RConn3 -- PS-Simulink Converter9/LConn1
  joint2/RConn3 -- PS-Simulink Converter10/LConn1
  joint3/RConn3 -- PS-Simulink Converter11/LConn1
  joint4/RConn3 -- PS-Simulink Converter12/LConn1
  joint5/RConn3 -- PS-Simulink Converter13/LConn1
  joint6/RConn3 -- PS-Simulink Converter14/LConn1

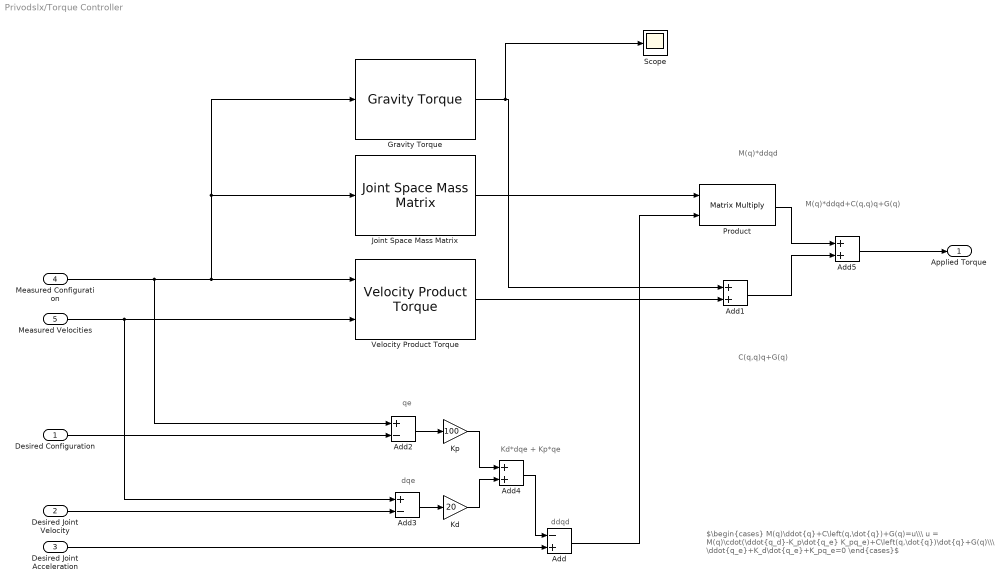
== system Privodslx/Torque Controller ==
  note: M(q)*ddqd+C(q,q)q+G(q)
  note: Kd*dqe + Kp*qe
  note: ddqd
  note: $\begin{cases} M(q)\ddot{q}+C\left(q,\dot{q})+G(q)=u\\\ u = M(q)\cdot(\ddot{q_d}-K_p\dot{q_e} K_pq_e)+C\left(q,\dot{q})\dot{q}+G(q)\\\ \ddot{q_e}+K_d\dot{q_e}+K_pq_e=0 \end{cases}$
  note: qe
  note: dqe
  note: C(q,q)q+G(q)
  note: M(q)*ddqd
  Desired Configuration : Inport  SampleTime=ts
  Desired Joint Velocity : Inport  Port=2  SampleTime=ts
  Desired Joint Acceleration : Inport  Port=3  SampleTime=ts
  Measured Configuration : Inport  Port=4  SampleTime=ts
  Measured Velocities : Inport  Port=5  SampleTime=ts
  Add : Sum  Inputs=-+
  Add1 : Sum
  Add2 : Sum  Inputs=+-
  Add3 : Sum  Inputs=+-
  Add4 : Sum
  Add5 : Sum
  Gravity Torque : robotmaniplib/Gravity Torque  RigidBodyTree=robot  SimulateUsing=Interpreted execution
  Joint Space Mass Matrix : robotmaniplib/Joint Space Mass Matrix  RigidBodyTree=robot  SimulateUsing=Interpreted execution
      settings: SourceProductName=Robotics System Toolbox
  Kd : Gain  Gain=20
  Kp : Gain  Gain=100
  Product : Product  Multiplication=Matrix(*)
  Scope : Scope
  Velocity Product Torque : robotmaniplib/Velocity Product Torque  RigidBodyTree=robot  SimulateUsing=Interpreted execution
      settings: SourceProductName=Robotics System Toolbox
  Applied Torque : Outport  SampleTime=ts  VectorParamsAs1DForOutWhenUnconnected=off
  wires:
  Desired Joint Acceleration/1 -> Add/2
  Desired Joint Velocity/1 -> Add3/2
  Desired Configuration/1 -> Add2/2
  Joint Space Mass Matrix/1 -> Product/1
  Measured Configuration/1 -> Gravity Torque/1, Joint Space Mass Matrix/1, Velocity Product Torque/1, Add2/1
  Measured Velocities/1 -> Add3/1, Velocity Product Torque/2
  Add4/1 -> Add/1
  Add3/1 -> Kd/1
  Kd/1 -> Add4/2
  Product/1 -> Add5/1
  Add1/1 -> Add5/2
  Gravity Torque/1 -> Scope/1, Add1/1
  Velocity Product Torque/1 -> Add1/2
  Add5/1 -> Applied Torque/1
  Kp/1 -> Add4/1
  Add2/1 -> Kp/1
  Add/1 -> Product/2

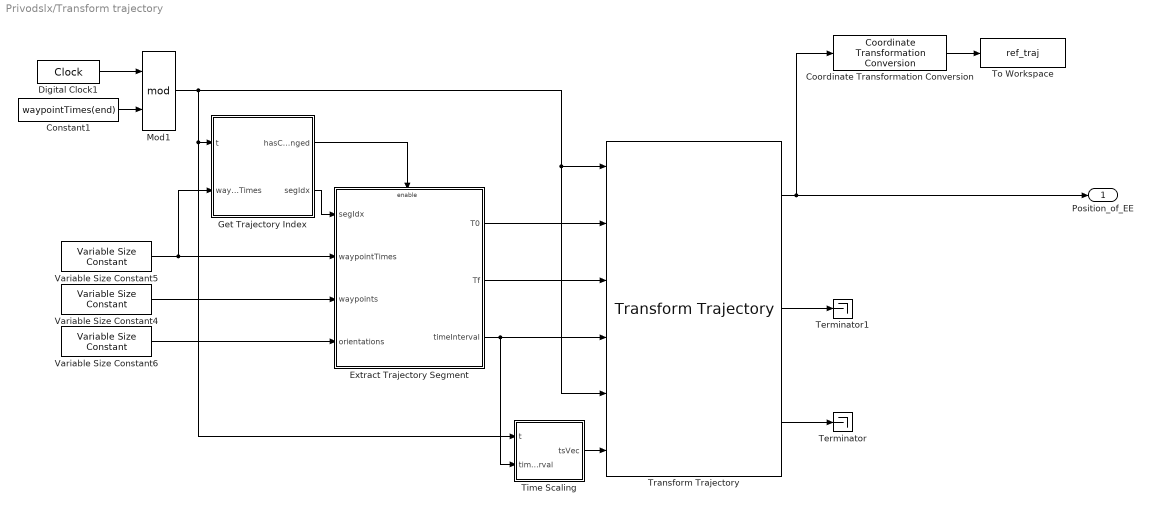
== system Privodslx/Transform trajectory ==
  Constant1 : Constant  Value=waypointTimes(end)  SampleTime=ts
  Coordinate Transformation Conversion : robotcorelib/Coordinate Transformation Conversion  InputRepresentation=Homogeneous Transformation  InputEulerSequence=ZYX  ShowTrVecInputPort=on  OutputRepresentation=Translation Vector  OutputEulerSequence=ZYX  ShowTrVecOutputPort=on  SimulateUsing=Interpreted execution
      settings: SourceProductBaseCode=RO,NV,RR,UV
  Digital Clock1 : DigitalClock  SampleTime=ts
  Extract Trajectory Segment : Subsystem
  Get Trajectory Index : MATLAB Function  TreatAsAtomicUnit=on
  Mod1 : Math  Operator=mod  SignedPower=on
  Terminator : Terminator
  Terminator1 : Terminator
  Time Scaling : Subsystem
  To Workspace : ToWorkspace  VariableName=ref_traj  SaveFormat=Timeseries  SampleTime=-1
  Transform Trajectory : robotcorelib/Transform Trajectory  WaypointSource=External  T0=trvec2tform( [ 1, 10, -1 ] )  TF=eul2tform( [ 0, pi, pi / 2 ] )  TimeInterval=[ 2, 3 ]  CustomTimeScaling=on  ParameterSource=External  TSTime=2:0.1:3  TimeScaling=[ 0:0.1:1; ones( 1, 11 ); zeros( 1, 11 ) ]  SimulateUsing=Interpreted execution
      settings: SourceProductBaseCode=RO,NV,RR,UV
  Variable Size Constant4 : trajExampleUtils/Variable Size Constant  val=waypoints  maxSize=[3,maxWaypoints]  Ts=ts  SSRTWFcnClass=[]
  Variable Size Constant5 : trajExampleUtils/Variable Size Constant  val=waypointTimes  maxSize=[1,maxWaypoints]  Ts=ts  SSRTWFcnClass=[]
  Variable Size Constant6 : trajExampleUtils/Variable Size Constant  val=orientations  maxSize=[3,maxWaypoints]  Ts=ts  SSRTWFcnClass=[]
  "Position_of_EE " : Outport  SampleTime=ts
  wires:
  Variable Size Constant5/1 -> Extract Trajectory Segment/2(waypointTimes), Get Trajectory Index/2(waypointTimes)
  Transform Trajectory/1 -> "Position_of_EE "/1, Coordinate Transformation Conversion/1
  Mod1/1 -> Transform Trajectory/5, Transform Trajectory/1, Time Scaling/1(t), Get Trajectory Index/1(t)
  Time Scaling/1(tsVec) -> Transform Trajectory/6
  Get Trajectory Index/2(segIdx) -> Extract Trajectory Segment/1(segIdx)
  Get Trajectory Index/1(hasChanged) -> Extract Trajectory Segment/Enable
  Extract Trajectory Segment/3(timeInterval) -> Transform Trajectory/4, Time Scaling/2(timeInterval)
  Constant1/1 -> Mod1/2
  Transform Trajectory/3 -> Terminator/1
  Extract Trajectory Segment/1(T0) -> Transform Trajectory/2
  Extract Trajectory Segment/2(Tf) -> Transform Trajectory/3
  Variable Size Constant4/1 -> Extract Trajectory Segment/3(waypoints)
  Transform Trajectory/2 -> Terminator1/1
  Variable Size Constant6/1 -> Extract Trajectory Segment/4(orientations)
  Digital Clock1/1 -> Mod1/1
  Coordinate Transformation Conversion/1 -> To Workspace/1

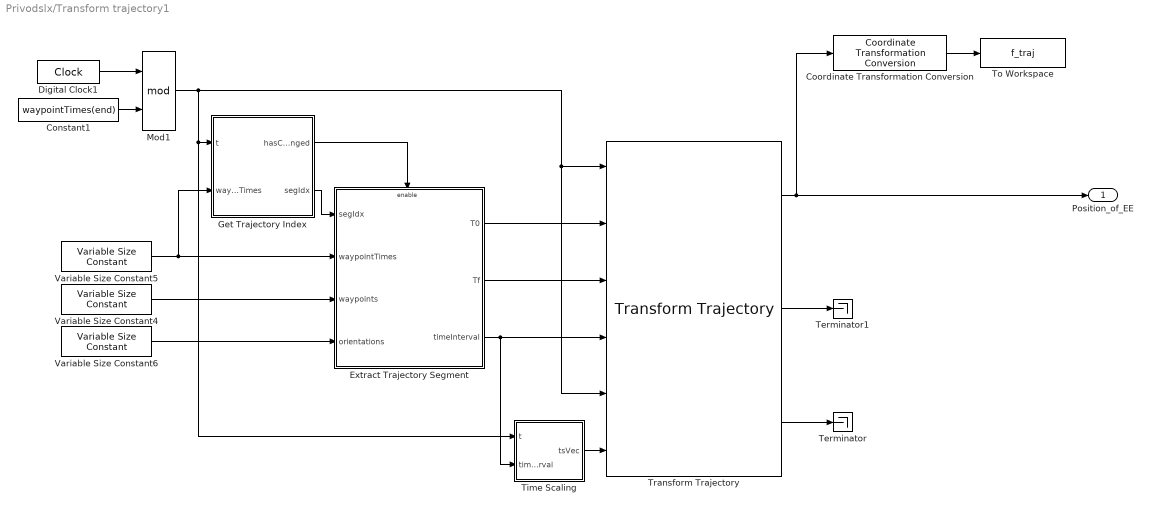
== system Privodslx/Transform trajectory1 ==
  Constant1 : Constant  Value=waypointTimes(end)
  Coordinate Transformation Conversion : robotcorelib/Coordinate Transformation Conversion  InputRepresentation=Homogeneous Transformation  InputEulerSequence=ZYX  ShowTrVecInputPort=on  OutputRepresentation=Translation Vector  OutputEulerSequence=ZYX  ShowTrVecOutputPort=on  SimulateUsing=Interpreted execution
      settings: SourceProductBaseCode=RO,NV,RR,UV
  Digital Clock1 : DigitalClock  SampleTime=ts
  Extract Trajectory Segment : Subsystem
  Get Trajectory Index : MATLAB Function  TreatAsAtomicUnit=on
  Mod1 : Math  Operator=mod  SignedPower=on
  Terminator : Terminator
  Terminator1 : Terminator
  Time Scaling : Subsystem
  To Workspace : ToWorkspace  VariableName=f_traj  SaveFormat=Timeseries  SampleTime=-1
  Transform Trajectory : robotcorelib/Transform Trajectory  WaypointSource=External  T0=trvec2tform( [ 1, 10, -1 ] )  TF=eul2tform( [ 0, pi, pi / 2 ] )  TimeInterval=[ 2, 3 ]  CustomTimeScaling=on  ParameterSource=External  TSTime=2:0.1:3  TimeScaling=[ 0:0.1:1; ones( 1, 11 ); zeros( 1, 11 ) ]  SimulateUsing=Interpreted execution
      settings: SourceProductBaseCode=RO,NV,RR,UV
  Variable Size Constant4 : trajExampleUtils/Variable Size Constant  val=waypoints  maxSize=[3,maxWaypoints]  Ts=-1
  Variable Size Constant5 : trajExampleUtils/Variable Size Constant  val=waypointTimes  maxSize=[1,maxWaypoints]  Ts=-1
  Variable Size Constant6 : trajExampleUtils/Variable Size Constant  val=orientations  maxSize=[3,maxWaypoints]  Ts=-1
  "Position_of_EE " : Outport
  wires:
  Coordinate Transformation Conversion/1 -> To Workspace/1
  Digital Clock1/1 -> Mod1/1
  Variable Size Constant6/1 -> Extract Trajectory Segment/4(orientations)
  Transform Trajectory/2 -> Terminator1/1
  Variable Size Constant4/1 -> Extract Trajectory Segment/3(waypoints)
  Extract Trajectory Segment/2(Tf) -> Transform Trajectory/3
  Extract Trajectory Segment/1(T0) -> Transform Trajectory/2
  Transform Trajectory/3 -> Terminator/1
  Constant1/1 -> Mod1/2
  Extract Trajectory Segment/3(timeInterval) -> Time Scaling/2(timeInterval), Transform Trajectory/4
  Get Trajectory Index/1(hasChanged) -> Extract Trajectory Segment/Enable
  Get Trajectory Index/2(segIdx) -> Extract Trajectory Segment/1(segIdx)
  Time Scaling/1(tsVec) -> Transform Trajectory/6
  Mod1/1 -> Get Trajectory Index/1(t), Time Scaling/1(t), Transform Trajectory/5, Transform Trajectory/1
  Transform Trajectory/1 -> Coordinate Transformation Conversion/1, "Position_of_EE "/1
  Variable Size Constant5/1 -> Get Trajectory Index/2(waypointTimes), Extract Trajectory Segment/2(waypointTimes)

== system Privodslx/Trapezoidal trajectory ==
  Constant5 : Constant  Value=waypointTimes(end)
  Coordinate Transformation Conversion : robotcorelib/Coordinate Transformation Conversion  InputRepresentation=Translation Vector  InputEulerSequence=ZYX  ShowTrVecInputPort=on  OutputRepresentation=Homogeneous Transformation  OutputEulerSequence=ZYX  ShowTrVecOutputPort=on  SimulateUsing=Interpreted execution
  Digital Clock : DigitalClock  SampleTime=ts
  Mod : Math  Operator=mod  SignedPower=on
  Polynomial Trajectory : robotcorelib/Polynomial Trajectory  WaypointSource=External  Waypoints=waypoints  TimePoints=[ 0, 1, 2,3,4,5,6]  TimeInterval=[ 1, 4 ]  Method=Cubic Polynomial  ParameterSource=External  VelocityBoundaryCondition=zeros( 3, 7 )  AccelerationBoundaryCondition=zeros( 2, 5 )  SimulateUsing=Interpreted execution
      settings: SourceProductBaseCode=RO,NV,RR,UV
  Terminator : Terminator
  Terminator1 : Terminator
  To Workspace : ToWorkspace  VariableName=f_traj  SaveFormat=Timeseries  SampleTime=-1
  Variable Size Constant : trajExampleUtils/Variable Size Constant  val=waypoints  maxSize=[3,maxWaypoints]  Ts=-1  SSRTWFcnClass=[]
  Variable Size Constant1 : trajExampleUtils/Variable Size Constant  val=waypointTimes  maxSize=[1,maxWaypoints]  Ts=-1  SSRTWFcnClass=[]
  Variable Size Constant2 : trajExampleUtils/Variable Size Constant  val=waypointVels  maxSize=[3,maxWaypoints]  Ts=-1  SSRTWFcnClass=[]
  Variable Size Constant3 : trajExampleUtils/Variable Size Constant  Commented=on  val=waypointAccels  maxSize=[3,maxWaypoints]  Ts=-1  SSRTWFcnClass=[]
  "Position_of_EE " : Outport
  wires:
  Digital Clock/1 -> Mod/1
  Polynomial Trajectory/1 -> To Workspace/1, Coordinate Transformation Conversion/1
  Polynomial Trajectory/2 -> Terminator/1
  Mod/1 -> Polynomial Trajectory/1
  Polynomial Trajectory/3 -> Terminator1/1
  Constant5/1 -> Mod/2
  Coordinate Transformation Conversion/1 -> "Position_of_EE "/1
  Variable Size Constant/1 -> Polynomial Trajectory/2
  Variable Size Constant1/1 -> Polynomial Trajectory/3
  Variable Size Constant2/1 -> Polynomial Trajectory/4

== system Privodslx/Trapezoidal trajectory1 ==
  Constant5 : Constant  Value=waypointTimes(end)
  Digital Clock : DigitalClock  SampleTime=ts
  Mod : Math  Operator=mod  SignedPower=on
  Polynomial Trajectory : robotcorelib/Polynomial Trajectory  WaypointSource=External  Waypoints=[ 0, 2, 1, 5, 0; -1, 3, 1, 4, 4 ]  TimePoints=[ 0, 1, 2, 3, 4 ]  TimeInterval=[ 1, 4 ]  Method=Quintic Polynomial  ParameterSource=External  VelocityBoundaryCondition=zeros( 2, 5 )  AccelerationBoundaryCondition=zeros( 2, 5 )  SimulateUsing=Interpreted execution
      settings: SourceProductBaseCode=RO,NV,RR,UV
  Variable Size Constant : trajExampleUtils/Variable Size Constant  val=waypoints  maxSize=[3,maxWaypoints]  Ts=-1
  Variable Size Constant1 : trajExampleUtils/Variable Size Constant  val=waypointTimes  maxSize=[1,maxWaypoints]  Ts=-1
  Variable Size Constant2 : trajExampleUtils/Variable Size Constant  val=waypointVels  maxSize=[3,maxWaypoints]  Ts=-1
  Variable Size Constant3 : trajExampleUtils/Variable Size Constant  val=waypointAccels  maxSize=[3,maxWaypoints]  Ts=-1
  q : Outport
  qd : Outport  Port=2
  qdd : Outport  Port=3
  wires:
  Constant5/1 -> Mod/2
  Variable Size Constant3/1 -> Polynomial Trajectory/5
  Variable Size Constant/1 -> Polynomial Trajectory/2
  Polynomial Trajectory/3 -> qdd/1
  Mod/1 -> Polynomial Trajectory/1
  Polynomial Trajectory/2 -> qd/1
  Polynomial Trajectory/1 -> q/1
  Variable Size Constant1/1 -> Polynomial Trajectory/3
  Variable Size Constant2/1 -> Polynomial Trajectory/4
  Digital Clock/1 -> Mod/1
